simulink model "TankBController"  (Simulink 8.1)
settings: Solver=ode45  StartTime=0.0  StopTime=10.0  RelTol=1e-3
settings Model: Creator=root  LastModifiedBy=root
settings DataIOCC: SignalLoggingSaveFormat=Dataset
settings OptimizationCC: ExpressionDepthLimit=128
settings DebuggingCC: FcnCallInpInsideContextMsg=EnableAllAsError
settings GRTTargetCC: CombineOutputUpdateFcns=on  GRTInterface=off

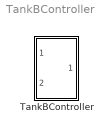
== system TankBController ==
  TankBController : Subsystem

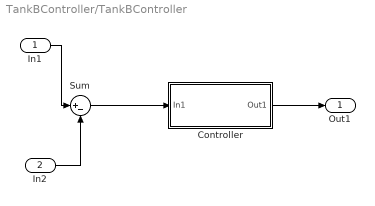
== system TankBController/TankBController ==
  In1 : Inport  OutDataTypeStr=double
  In2 : Inport  Port=2  OutDataTypeStr=double
  Controller : Subsystem
  Sum : Sum  Inputs=|+-
  Out1 : Outport  OutDataTypeStr=double
  wires:
  In2/1 -> Sum/2
  In1/1 -> Sum/1
  Controller/1(Out1) -> Out1/1
  Sum/1 -> Controller/1(In1)

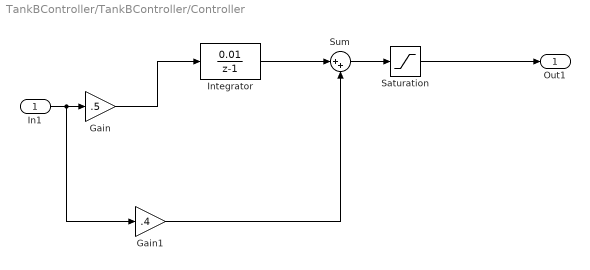
== system TankBController/TankBController/Controller ==
  In1 : Inport
  Gain : Gain  Gain=.5
  Gain1 : Gain  Gain=.4
  Integrator : DiscreteTransferFcn  Numerator=[0.01]  Denominator=[1 -1]  SampleTime=0.01
  Saturation : Saturate  UpperLimit=10  LowerLimit=0
  Sum : Sum  Inputs=|++
  Out1 : Outport
  wires:
  Saturation/1 -> Out1/1
  In1/1 -> Gain1/1, Gain/1
  Gain/1 -> Integrator/1
  Gain1/1 -> Sum/2
  Integrator/1 -> Sum/1
  Sum/1 -> Saturation/1
